simulink library "two_axis_control_lib"  (R2016b)
settings: Solver=VariableStepAuto  StartTime=0.0  StopTime=10.0  RelTol=1e-3
undefined symbols (not defined in the file or in its folder): K1, K2
libraries: aerolibutil x3
settings Model: Creator=unsik  LastModifiedBy=unsik

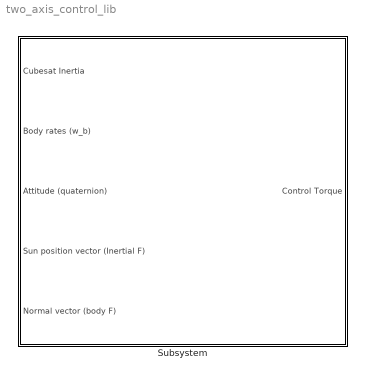
== system two_axis_control_lib ==
  Subsystem : Subsystem

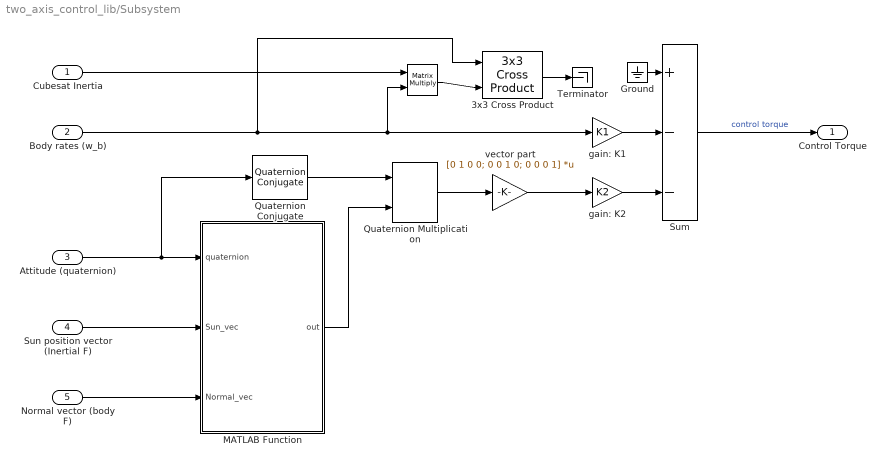
== system two_axis_control_lib/Subsystem ==
  Cubesat Inertia : Inport
  Body rates (w_b) : Inport  Port=2
  Attitude (quaternion) : Inport  Port=3
  Sun position vector (Inertial F) : Inport  Port=4
  Normal vector (body F) : Inport  Port=5
  " " : Product  Multiplication=Matrix(*)
  3x3 Cross Product : aerolibutil/3x3 Cross Product
  Ground : Ground
  MATLAB Function : MATLAB Function  TreatAsAtomicUnit=on
  Quaternion Conjugate : aerolibutil/Quaternion Conjugate
  Quaternion Multiplication : aerolibutil/Quaternion Multiplication
  Sum : Sum  Inputs=+--
  Terminator : Terminator
  gain: K1 : Gain  Gain=K1
  gain: K2 : Gain  Gain=K2
  vector part : Gain  Gain=[0 1 0 0; 0 0 1 0; 0 0 0 1]  Multiplication=Matrix(K*u)
  Control Torque : Outport
  wires:
  Sun position vector (Inertial F)/1 -> MATLAB Function/2(Sun_vec)
  Attitude (quaternion)/1 -> Quaternion Conjugate/1, MATLAB Function/1(quaternion)
  Quaternion Conjugate/1 -> Quaternion Multiplication/1
  MATLAB Function/1(out) -> Quaternion Multiplication/2
  Quaternion Multiplication/1 -> vector part/1
  Cubesat Inertia/1 -> " "/1
  Body rates (w_b)/1 -> 3x3 Cross Product/1, " "/2, gain: K1/1
  vector part/1 -> gain: K2/1
  Sum/1 -> Control Torque/1  "control torque"
  Normal vector (body F)/1 -> MATLAB Function/3(Normal_vec)
  gain: K1/1 -> Sum/2
  " "/1 -> 3x3 Cross Product/2
  gain: K2/1 -> Sum/3
  3x3 Cross Product/1 -> Terminator/1
  Ground/1 -> Sum/1

== matlab function two_axis_control_lib/Subsystem/MATLAB Function ==
  data: quaternion input; Sun_vec input; out output; Normal_vec input
function out = fcn(quaternion,Sun_vec, Normal_vec)
% sun position vector in Inertial frame
Sx = Sun_vec(1);
Sy = Sun_vec(2);
Sz = Sun_vec(3);

% solar panel normal vector in Body frame
Bx = Normal_vec(1);
By = Normal_vec(2);
Bz = Normal_vec(3);

M = [1-By*Sy-Bz*Sz-Bx*Sx, Bz*Sy-By*Sz, Bx*Sz - Bz*Sx, By*Sx-Bx*Sy; 
     Bz*Sy-By*Sz, By*Sy-Bx*Sx+Bz*Sz+1, -Bx*Sy-By*Sx, -Bx*Sz-Bz*Sx; 
     Bx*Sz-Bz*Sx, -Bx*Sy-By*Sx, Bx*Sx-By*Sy+Bz*Sz+1, -By*Sz-Bz*Sy; 
     By*Sx-Bx*Sy, -Bx*Sz-Bz*Sx, -By*Sz-Bz*Sy, Bx*Sx+By*Sy-Bz*Sz+1];

out = 2*M*quaternion;
